simulink model "cubli_XYZ_extensive_simulations"  (R2016a)
settings: Solver=VariableStepAuto  StartTime=0.0  StopTime=10  FixedStep=0.001  RelTol=1e-3
values from neighbouring files (symbols this model uses):
  a = 0.15    [init.m]
  M = 2.5    [init.m]    (also in skew.m = [0 -z y)
  m = 0.204    [init.m]
  s = size(delta_i)    [accessibility_test.m]    (also in observability_test.m = size(delta_i,1))
  state0 = get_equilibrium(0, -pi/4, pi/2, f, state)    [init.m]
undefined symbols (not defined in the file or in its folder): X, Y, Z
libraries: sm_lib x15, nesl_utility x13
(part 7 of 9)

== matlab function cubli_XYZ_extensive_simulations/Cubli/Controller/LQR at equilibrium ==
  data: state input; Q input; R input; u output; theta parameter; state0 parameter
 function u = nic_fnc(state, Q, R, theta, state0)

 %% persistent variables
persistent K_lqr state_eq

 %% lqr cannot be used AS IS in matlab functions
coder.extrinsic('lqr');
coder.extrinsic('ctrbf');

 %% initialize persistent variables
if isempty (K_lqr)
    K_lqr = zeros(3,9);
    state_eq = zeros(9,1);
    K = zeros(3,8);
    Aalt = zeros(9);
    Q_lqr = zeros(9);
    Balt = zeros(9,3);
    
    % equilibrium state
    state_eq = angles(theta, state0);
    
    % linearize around equilibrium
    th1 = state_eq(1);
    th2 = state_eq(2);
    th3 = state_eq(3);
    th1dot = state_eq(4);
    th2dot = state_eq(5);
    th3dot = state_eq(6);
    qxdot = state_eq(7);
    qydot = state_eq(8);
    qzdot = state_eq(9);
    u1 = 0;
    u2 = 0;
    u3 = 0;
    
    % evaluate A and B s.t. dx_dot = A * dx + B * du
    A = [
         0, 0, 0, 1, 0, 0, 0, 0, 0
         0, 0, 0, 0, 1, 0, 0, 0, 0
         0, 0, 0, 0, 0, 1, 0, 0, 0
         (5234057499985498930356104062315637394898944*cos(th1) + 5234057499985498930356104062315637394898944*cos(th2)*sin(th1)*sin(th3) + 5234057499985498930356104062315637394898944*cos(th2)*cos(th3)*sin(th1))/(140800205444266547517405832452217960942325*cos(th2)),                                                                                                                                                                                                                                                                                                                                                                                                                                                                                                                                                                                                                                                                                                                                                                                                                                                                                                                                                                                                                                                                                                                                                                                                                                                                                                                                                                                                                                                                                                                                                                                                                                                                                                                                                                                                                                                                                                                                                                                                                                                                                                                                                                                                                                                                                                                                                                                                                                                                                                                                                                                                                                                                                                                                                                                                                                                                                                                                                                                                                                                                                                                                                                                                                                                                                                                                                                                                                                                                                                                                                                                                                                                                                                                                                                                                                                                                                                                                                                                                                                                                                                                                                                                                                                                                                                                                                                                                                                                                                                                                                                                                                                                                                                                                                                                                                                                                                                                                                                                          (37208574363983751213784670214039629987840*th1dot^2*cos(2*th2) + 5234057499985498930356104062315637394898944*cos(th1)*sin(th2)*sin(th3) + 140800205444266547517405832452217960942325*th1dot*th2dot*cos(th2) - 795598339977096578581794905915392000000*qxdot*th1dot*sin(th2) + 795598339977096578581794905915392000000*qzdot*th1dot*sin(th2) - 37208574363983751213784670214039629987840*th1dot*th3dot*sin(th2) - 74417148727967502427569340428079259975680*th1dot^2*cos(th2)^2*cos(th3)^2 + 74417148727967502427569340428079259975680*th1dot^2*cos(th3)^2*sin(th2)^2 + 5234057499985498930356104062315637394898944*cos(th1)*cos(th3)*sin(th2) + 1419410730694772925795933922925238500000*qxdot*th1dot*cos(th2)*sin(th3) - 795598339977096578581794905915392000000*qydot*th1dot*cos(th2)*sin(th3) - 37208574363983751213784670214039629987840*th1dot*th2dot*cos(th3)*sin(th2) - 74417148727967502427569340428079259975680*th1dot*th3dot*cos(th2)*sin(th3) + 37208574363983751213784670214039629987840*th1dot*th2dot*sin(th2)*sin(th3) + 795598339977096578581794905915392000000*qxdot*th1dot*cos(th3)^2*sin(th2) + 795598339977096578581794905915392000000*qydot*th1dot*cos(th3)^2*sin(th2) - 1591196679954193157163589811830784000000*qzdot*th1dot*cos(th3)^2*sin(th2) + 74417148727967502427569340428079259975680*th1dot*th3dot*cos(th3)^2*sin(th2) - 74417148727967502427569340428079259975680*th1dot^2*cos(th2)*cos(th3)*sin(th2) - 74417148727967502427569340428079259975680*th1dot^2*cos(th2)*sin(th2)*sin(th3) - 795598339977096578581794905915392000000*qxdot*th1dot*cos(th2)*cos(th3) + 1419410730694772925795933922925238500000*qydot*th1dot*cos(th2)*cos(th3) - 74417148727967502427569340428079259975680*th1dot*th3dot*cos(th2)*cos(th3) - 74417148727967502427569340428079259975680*th1dot*th2dot*cos(th2)*cos(th3)*sin(th3) + 795598339977096578581794905915392000000*qxdot*th1dot*cos(th3)*sin(th2)*sin(th3) - 795598339977096578581794905915392000000*qydot*th1dot*cos(th3)*sin(th2)*sin(th3))/(140800205444266547517405832452217960942325*cos(th2)) - (sin(th2)*(37208574363983751213784670214039629987840*th1dot^2*cos(th3) - 5234057499985498930356104062315637394898944*sin(th1) - 37208574363983751213784670214039629987840*th2dot^2*cos(th3) + 37208574363983751213784670214039629987840*th3dot^2*cos(th3) + 37208574363983751213784670214039629987840*th1dot^2*sin(th3) - 37208574363983751213784670214039629987840*th2dot^2*sin(th3) + 37208574363983751213784670214039629987840*th3dot^2*sin(th3) - 795598339977096578581794905915392000000*qydot*th2dot + 1419410730694772925795933922925238500000*qzdot*th2dot + 140800205444266547517405832452217960942325*th2dot*th3dot - 18604287181991875606892335107019814993920*th1dot^2*sin(2*th2) - 795598339977096578581794905915392000000*qxdot*th1dot*cos(th2) + 795598339977096578581794905915392000000*qxdot*th3dot*cos(th3) - 1419410730694772925795933922925238500000*qydot*th3dot*cos(th3) + 795598339977096578581794905915392000000*qzdot*th1dot*cos(th2) - 37208574363983751213784670214039629987840*th1dot*th3dot*cos(th2) - 1419410730694772925795933922925238500000*qxdot*th3dot*sin(th3) + 795598339977096578581794905915392000000*qydot*th3dot*sin(th3) - 140800205444266547517405832452217960942325*th1dot*th2dot*sin(th2) - 37208574363983751213784670214039629987840*th1dot^2*cos(th2)^2*cos(th3) - 37208574363983751213784670214039629987840*th1dot^2*cos(th2)^2*sin(th3) - 795598339977096578581794905915392000000*qxdot*th2dot*cos(th3)^2 + 795598339977096578581794905915392000000*qydot*th2dot*cos(th3)^2 + 397799169988548289290897452957696000000*qxdot*th2dot*sin(2*th3) + 397799169988548289290897452957696000000*qydot*th2dot*sin(2*th3) - 795598339977096578581794905915392000000*qzdot*th2dot*sin(2*th3) + 37208574363983751213784670214039629987840*th2dot*th3dot*sin(2*th3) + 5234057499985498930356104062315637394898944*cos(th1)*cos(th2)*cos(th3) + 5234057499985498930356104062315637394898944*cos(th1)*cos(th2)*sin(th3) + 795598339977096578581794905915392000000*qxdot*th1dot*cos(th3)*sin(th2) - 1419410730694772925795933922925238500000*qydot*th1dot*cos(th3)*sin(th2) + 37208574363983751213784670214039629987840*th1dot*th2dot*cos(th2)*sin(th3) + 74417148727967502427569340428079259975680*th1dot*th3dot*cos(th3)*sin(th2) - 1419410730694772925795933922925238500000*qxdot*th1dot*sin(th2)*sin(th3) + 795598339977096578581794905915392000000*qydot*th1dot*sin(th2)*sin(th3) + 74417148727967502427569340428079259975680*th1dot*th3dot*sin(th2)*sin(th3) + 74417148727967502427569340428079259975680*th1dot^2*cos(th2)*cos(th3)^2*sin(th2) + 795598339977096578581794905915392000000*qxdot*th1dot*cos(th2)*cos(th3)^2 + 795598339977096578581794905915392000000*qydot*th1dot*cos(th2)*cos(th3)^2 - 1591196679954193157163589811830784000000*qzdot*th1dot*cos(th2)*cos(th3)^2 + 74417148727967502427569340428079259975680*th1dot*th3dot*cos(th2)*cos(th3)^2 - 37208574363983751213784670214039629987840*th1dot*th2dot*cos(th2)*cos(th3) + 795598339977096578581794905915392000000*qxdot*th1dot*cos(th2)*cos(th3)*sin(th3) - 795598339977096578581794905915392000000*qydot*th1dot*cos(th2)*cos(th3)*sin(th3) + 74417148727967502427569340428079259975680*th1dot*th2dot*cos(th3)*sin(th2)*sin(th3)))/(140800205444266547517405832452217960942325*cos(th2)^2) - (11529215046068469760000*u1*sin(th2)*(173808361171031714041*cos(th3) - 97421867139278569472*sin(th3)))/(50688073959935957106266099682798465939237*cos(th2)^2) - (11529215046068469760000*u2*sin(th2)*(97421867139278569472*cos(th3) - 173808361171031714041*sin(th3)))/(50688073959935957106266099682798465939237*cos(th2)^2) - (1123197656438253912603716965936891166720000*2^(1/2)*u3*cos(th3 + pi/4)*sin(th2))/(50688073959935957106266099682798465939237*cos(th2)^2),                                                                                                                                                                                                                                                                                                                                                                                                                                                                                                                                                                                                                                                                                                                                                                                                                                                                                                                                                                                                                                                                                                                                                                                                                                                                                                                                                                                                                                                                                                                    (11529215046068469760000*u1*(97421867139278569472*cos(th3) + 173808361171031714041*sin(th3)))/(50688073959935957106266099682798465939237*cos(th2)) - (37208574363983751213784670214039629987840*th1dot^2*cos(th3) - 37208574363983751213784670214039629987840*th2dot^2*cos(th3) + 37208574363983751213784670214039629987840*th3dot^2*cos(th3) - 37208574363983751213784670214039629987840*th1dot^2*sin(th3) + 37208574363983751213784670214039629987840*th2dot^2*sin(th3) - 37208574363983751213784670214039629987840*th3dot^2*sin(th3) - 1419410730694772925795933922925238500000*qxdot*th3dot*cos(th3) + 795598339977096578581794905915392000000*qydot*th3dot*cos(th3) - 795598339977096578581794905915392000000*qxdot*th3dot*sin(th3) + 1419410730694772925795933922925238500000*qydot*th3dot*sin(th3) - 37208574363983751213784670214039629987840*th1dot^2*cos(th2)^2*cos(th3) + 37208574363983751213784670214039629987840*th1dot^2*cos(th2)^2*sin(th3) + 795598339977096578581794905915392000000*qxdot*th2dot*cos(2*th3) + 795598339977096578581794905915392000000*qydot*th2dot*cos(2*th3) - 1591196679954193157163589811830784000000*qzdot*th2dot*cos(2*th3) + 74417148727967502427569340428079259975680*th2dot*th3dot*cos(2*th3) + 5234057499985498930356104062315637394898944*cos(th1)*cos(th2)*cos(th3) - 5234057499985498930356104062315637394898944*cos(th1)*cos(th2)*sin(th3) - 1419410730694772925795933922925238500000*qxdot*th1dot*cos(th3)*sin(th2) + 1591196679954193157163589811830784000000*qxdot*th2dot*cos(th3)*sin(th3) + 795598339977096578581794905915392000000*qydot*th1dot*cos(th3)*sin(th2) - 1591196679954193157163589811830784000000*qydot*th2dot*cos(th3)*sin(th3) + 37208574363983751213784670214039629987840*th1dot*th2dot*cos(th2)*sin(th3) + 74417148727967502427569340428079259975680*th1dot*th3dot*cos(th3)*sin(th2) - 795598339977096578581794905915392000000*qxdot*th1dot*sin(th2)*sin(th3) + 1419410730694772925795933922925238500000*qydot*th1dot*sin(th2)*sin(th3) - 74417148727967502427569340428079259975680*th1dot*th3dot*sin(th2)*sin(th3) + 795598339977096578581794905915392000000*qxdot*th1dot*cos(th2)*cos(th3)^2 - 795598339977096578581794905915392000000*qydot*th1dot*cos(th2)*cos(th3)^2 - 795598339977096578581794905915392000000*qxdot*th1dot*cos(th2)*sin(th3)^2 + 795598339977096578581794905915392000000*qydot*th1dot*cos(th2)*sin(th3)^2 + 74417148727967502427569340428079259975680*th1dot*th2dot*cos(th3)^2*sin(th2) - 74417148727967502427569340428079259975680*th1dot*th2dot*sin(th2)*sin(th3)^2 + 37208574363983751213784670214039629987840*th1dot*th2dot*cos(th2)*cos(th3) - 148834297455935004855138680856158519951360*th1dot^2*cos(th2)*cos(th3)*sin(th2)*sin(th3) - 1591196679954193157163589811830784000000*qxdot*th1dot*cos(th2)*cos(th3)*sin(th3) - 1591196679954193157163589811830784000000*qydot*th1dot*cos(th2)*cos(th3)*sin(th3) + 3182393359908386314327179623661568000000*qzdot*th1dot*cos(th2)*cos(th3)*sin(th3) - 148834297455935004855138680856158519951360*th1dot*th3dot*cos(th2)*cos(th3)*sin(th3))/(140800205444266547517405832452217960942325*cos(th2)) + (11529215046068469760000*u2*(173808361171031714041*cos(th3) + 97421867139278569472*sin(th3)))/(50688073959935957106266099682798465939237*cos(th2)) + (1123197656438253912603716965936891166720000*2^(1/2)*u3*sin(th3 + pi/4))/(50688073959935957106266099682798465939237*cos(th2)),                                                                                                                                                                                                                                                                                                                                                                                                                                 -(795598339977096578581794905915392000000*qzdot*cos(th2) - 795598339977096578581794905915392000000*qxdot*cos(th2) - 37208574363983751213784670214039629987840*th1dot*sin(2*th2) + 74417148727967502427569340428079259975680*th1dot*cos(th3) - 37208574363983751213784670214039629987840*th3dot*cos(th2) + 74417148727967502427569340428079259975680*th1dot*sin(th3) - 140800205444266547517405832452217960942325*th2dot*sin(th2) - 37208574363983751213784670214039629987840*th2dot*cos(th2)*cos(th3) + 795598339977096578581794905915392000000*qxdot*cos(th3)*sin(th2) - 1419410730694772925795933922925238500000*qydot*cos(th3)*sin(th2) + 37208574363983751213784670214039629987840*th2dot*cos(th2)*sin(th3) + 74417148727967502427569340428079259975680*th3dot*cos(th3)*sin(th2) - 1419410730694772925795933922925238500000*qxdot*sin(th2)*sin(th3) + 795598339977096578581794905915392000000*qydot*sin(th2)*sin(th3) + 74417148727967502427569340428079259975680*th3dot*sin(th2)*sin(th3) + 795598339977096578581794905915392000000*qxdot*cos(th2)*cos(th3)^2 + 795598339977096578581794905915392000000*qydot*cos(th2)*cos(th3)^2 - 1591196679954193157163589811830784000000*qzdot*cos(th2)*cos(th3)^2 - 74417148727967502427569340428079259975680*th1dot*cos(th2)^2*cos(th3) + 74417148727967502427569340428079259975680*th3dot*cos(th2)*cos(th3)^2 - 74417148727967502427569340428079259975680*th1dot*cos(th2)^2*sin(th3) + 795598339977096578581794905915392000000*qxdot*cos(th2)*cos(th3)*sin(th3) - 795598339977096578581794905915392000000*qydot*cos(th2)*cos(th3)*sin(th3) + 74417148727967502427569340428079259975680*th2dot*cos(th3)*sin(th2)*sin(th3) + 148834297455935004855138680856158519951360*th1dot*cos(th2)*cos(th3)^2*sin(th2))/(140800205444266547517405832452217960942325*cos(th2)),                                                                                                                                                                                                                                                                                                                                                                                                                                                                                                                                                                                                                                                                                                                                                                 -(1419410730694772925795933922925238500000*qzdot - 795598339977096578581794905915392000000*qydot + 140800205444266547517405832452217960942325*th3dot - 795598339977096578581794905915392000000*qxdot*cos(th3)^2 + 795598339977096578581794905915392000000*qydot*cos(th3)^2 + 397799169988548289290897452957696000000*qxdot*sin(2*th3) + 397799169988548289290897452957696000000*qydot*sin(2*th3) - 795598339977096578581794905915392000000*qzdot*sin(2*th3) + 37208574363983751213784670214039629987840*th3dot*sin(2*th3) - 74417148727967502427569340428079259975680*th2dot*cos(th3) - 140800205444266547517405832452217960942325*th1dot*sin(th2) - 74417148727967502427569340428079259975680*th2dot*sin(th3) - 37208574363983751213784670214039629987840*th1dot*cos(th2)*cos(th3) + 37208574363983751213784670214039629987840*th1dot*cos(th2)*sin(th3) + 74417148727967502427569340428079259975680*th1dot*cos(th3)*sin(th2)*sin(th3))/(140800205444266547517405832452217960942325*cos(th2)),                                                                                                                                                                                                                                                                                                                                                                                                                                                                                  -(140800205444266547517405832452217960942325*th2dot + 37208574363983751213784670214039629987840*th2dot*sin(2*th3) + 795598339977096578581794905915392000000*qxdot*cos(th3) - 1419410730694772925795933922925238500000*qydot*cos(th3) - 37208574363983751213784670214039629987840*th1dot*cos(th2) + 74417148727967502427569340428079259975680*th3dot*cos(th3) - 1419410730694772925795933922925238500000*qxdot*sin(th3) + 795598339977096578581794905915392000000*qydot*sin(th3) + 74417148727967502427569340428079259975680*th3dot*sin(th3) + 74417148727967502427569340428079259975680*th1dot*cos(th3)*sin(th2) + 74417148727967502427569340428079259975680*th1dot*sin(th2)*sin(th3) + 74417148727967502427569340428079259975680*th1dot*cos(th2)*cos(th3)^2)/(140800205444266547517405832452217960942325*cos(th2)),                                                                                                                                                                                                                                                                                                                                -(397799169988548289290897452957696000000*th2dot*sin(2*th3) - 795598339977096578581794905915392000000*th2dot*cos(th3)^2 - 795598339977096578581794905915392000000*th1dot*cos(th2) + 795598339977096578581794905915392000000*th3dot*cos(th3) - 1419410730694772925795933922925238500000*th3dot*sin(th3) + 795598339977096578581794905915392000000*th1dot*cos(th3)*sin(th2) - 1419410730694772925795933922925238500000*th1dot*sin(th2)*sin(th3) + 795598339977096578581794905915392000000*th1dot*cos(th2)*cos(th3)^2 + 795598339977096578581794905915392000000*th1dot*cos(th2)*cos(th3)*sin(th3))/(140800205444266547517405832452217960942325*cos(th2)),                                                                                                                                                                                                                                                                                                                                -(795598339977096578581794905915392000000*th2dot*cos(th3)^2 - 795598339977096578581794905915392000000*th2dot + 397799169988548289290897452957696000000*th2dot*sin(2*th3) - 1419410730694772925795933922925238500000*th3dot*cos(th3) + 795598339977096578581794905915392000000*th3dot*sin(th3) - 1419410730694772925795933922925238500000*th1dot*cos(th3)*sin(th2) + 795598339977096578581794905915392000000*th1dot*sin(th2)*sin(th3) + 795598339977096578581794905915392000000*th1dot*cos(th2)*cos(th3)^2 - 795598339977096578581794905915392000000*th1dot*cos(th2)*cos(th3)*sin(th3))/(140800205444266547517405832452217960942325*cos(th2)),                                                                                                                                                                                                                                                                                                                     -(1419410730694772925795933922925238500000*th2dot - 795598339977096578581794905915392000000*th2dot*sin(2*th3) + 795598339977096578581794905915392000000*th1dot*cos(th2) - 1591196679954193157163589811830784000000*th1dot*cos(th2)*cos(th3)^2)/(140800205444266547517405832452217960942325*cos(th2))
         (68520719092170281189376*cos(th2)*sin(th1)*sin(th3))/1843260477247944264925 - (68520719092170281189376*sin(th1)*sin(th2))/1843260477247944264925 - (68520719092170281189376*cos(th2)*cos(th3)*sin(th1))/1843260477247944264925,                                                                                                                                                                                                                                                                                                                                                                                                                                                                                                                                                                                                                                                                                                                                                                                                                                                                                                                                                                                                                                                                                                                                                                                                                                                                                                                                                                                                                                                                                                                                                                                                                                                                                                                                                                                                                                                                                                                                                                                                                                                                                                                                                                                                                                                                                                                                                                                                                                                                                                                                                                                                                                                                                                                                                                                                                                                                                                                                                                                                                                                                                                                                                                                                                                                                                                                                                                                                                                                                                                                                                                                                                                                                                                                                                                                                                                                                                                                                                                                                                                                                                                                                                                                                                                                                                                                                                                                                                                                                                                                                                                                                                                                                                                                                                                                                                                                                                                                                                                                                                                                                                                                                                                                                                                                                                                                                                                                                                                                                                                                                                                                                                                                                                                                                                                                                                                                                                                                                                                                                                                                                                                                                                                                                                                                                                                                                                                                                                                                                                                                                                                                                                                                                                                                                                                                                                                                                                                                                                                                                                                                                                                                                                                                                                                                                                                                                                                                                                                                                                                                                                                                                                                                                                                                                                                                                                                                                                                                                                                                                                                                                                                                                                                                                                                                                                                                       (68520719092170281189376*cos(th1)*cos(th2))/1843260477247944264925 + (68520719092170281189376*cos(th1)*sin(th2)*sin(th3))/1843260477247944264925 - (97421867139278569472*th1dot*th2dot*cos(th2))/368652095449588852985 + (31823933599083863143271796236615680000*qxdot*th1dot*sin(th2))/5632008217770661900696233298088718437693 - (56776429227790917031837356917009540000*qzdot*th1dot*sin(th2))/5632008217770661900696233298088718437693 - th1dot*th3dot*sin(th2) - (68520719092170281189376*cos(th1)*cos(th3)*sin(th2))/1843260477247944264925 - (31823933599083863143271796236615680000*qxdot*th1dot*cos(th2)*sin(th3))/5632008217770661900696233298088718437693 + (56776429227790917031837356917009540000*qydot*th1dot*cos(th2)*sin(th3))/5632008217770661900696233298088718437693 + (97421867139278569472*th1dot*th2dot*cos(th3)*sin(th2))/368652095449588852985 - (194843734278557138944*th1dot*th3dot*cos(th2)*sin(th3))/368652095449588852985 + (97421867139278569472*th1dot*th2dot*sin(th2)*sin(th3))/368652095449588852985 - (194843734278557138944*th1dot^2*cos(th2)^2*cos(th3)*sin(th3))/368652095449588852985 + (194843734278557138944*th1dot^2*cos(th3)*sin(th2)^2*sin(th3))/368652095449588852985 + (194843734278557138944*th1dot*th2dot*cos(th2)*cos(th3)^2)/368652095449588852985 - (31823933599083863143271796236615680000*qxdot*th1dot*cos(th3)^2*sin(th2))/5632008217770661900696233298088718437693 + (31823933599083863143271796236615680000*qydot*th1dot*cos(th3)^2*sin(th2))/5632008217770661900696233298088718437693 + (389687468557114277888*th1dot^2*cos(th2)*cos(th3)*sin(th2))/368652095449588852985 - (389687468557114277888*th1dot^2*cos(th2)*sin(th2)*sin(th3))/368652095449588852985 - (56776429227790917031837356917009540000*qxdot*th1dot*cos(th2)*cos(th3))/5632008217770661900696233298088718437693 + (31823933599083863143271796236615680000*qydot*th1dot*cos(th2)*cos(th3))/5632008217770661900696233298088718437693 + (194843734278557138944*th1dot*th3dot*cos(th2)*cos(th3))/368652095449588852985 + (31823933599083863143271796236615680000*qxdot*th1dot*cos(th3)*sin(th2)*sin(th3))/5632008217770661900696233298088718437693 + (31823933599083863143271796236615680000*qydot*th1dot*cos(th3)*sin(th2)*sin(th3))/5632008217770661900696233298088718437693 - (63647867198167726286543592473231360000*qzdot*th1dot*cos(th3)*sin(th2)*sin(th3))/5632008217770661900696233298088718437693 + (194843734278557138944*th1dot*th3dot*cos(th3)*sin(th2)*sin(th3))/368652095449588852985,                                                                                                                                                                                                                                                                                                                                                                                                                                                               (56776429227790917031837356917009540000*qydot*th3dot*cos(th3))/5632008217770661900696233298088718437693 - (97421867139278569472*th3dot^2*cos(th3))/368652095449588852985 - u1*((2003873972745561633640040521298775900160000*cos(th3))/50688073959935957106266099682798465939237 - (1123197656438253912603716965936891166720000*sin(th3))/50688073959935957106266099682798465939237) - u2*((1123197656438253912603716965936891166720000*cos(th3))/50688073959935957106266099682798465939237 - (2003873972745561633640040521298775900160000*sin(th3))/50688073959935957106266099682798465939237) - (97421867139278569472*th1dot^2*sin(th3))/368652095449588852985 - (97421867139278569472*th3dot^2*sin(th3))/368652095449588852985 - (1123197656438253912603716965936891166720000*2^(1/2)*u3*cos(th3 + pi/4))/50688073959935957106266099682798465939237 - (31823933599083863143271796236615680000*qxdot*th3dot*cos(th3))/5632008217770661900696233298088718437693 - (97421867139278569472*th1dot^2*cos(th3))/368652095449588852985 + (56776429227790917031837356917009540000*qxdot*th3dot*sin(th3))/5632008217770661900696233298088718437693 - (31823933599083863143271796236615680000*qydot*th3dot*sin(th3))/5632008217770661900696233298088718437693 + (194843734278557138944*th1dot^2*cos(th2)^2*cos(th3))/368652095449588852985 + (194843734278557138944*th1dot^2*cos(th2)^2*sin(th3))/368652095449588852985 + (31823933599083863143271796236615680000*qxdot*th2dot*cos(2*th3))/5632008217770661900696233298088718437693 - (31823933599083863143271796236615680000*qydot*th2dot*cos(2*th3))/5632008217770661900696233298088718437693 - (68520719092170281189376*cos(th1)*cos(th2)*cos(th3))/1843260477247944264925 - (68520719092170281189376*cos(th1)*cos(th2)*sin(th3))/1843260477247944264925 - (31823933599083863143271796236615680000*qxdot*th1dot*cos(th3)*sin(th2))/5632008217770661900696233298088718437693 - (63647867198167726286543592473231360000*qxdot*th2dot*cos(th3)*sin(th3))/5632008217770661900696233298088718437693 + (56776429227790917031837356917009540000*qydot*th1dot*cos(th3)*sin(th2))/5632008217770661900696233298088718437693 - (63647867198167726286543592473231360000*qydot*th2dot*cos(th3)*sin(th3))/5632008217770661900696233298088718437693 + (127295734396335452573087184946462720000*qzdot*th2dot*cos(th3)*sin(th3))/5632008217770661900696233298088718437693 + (97421867139278569472*th1dot*th2dot*cos(th2)*sin(th3))/368652095449588852985 - (194843734278557138944*th1dot*th3dot*cos(th3)*sin(th2))/368652095449588852985 - (389687468557114277888*th2dot*th3dot*cos(th3)*sin(th3))/368652095449588852985 + (56776429227790917031837356917009540000*qxdot*th1dot*sin(th2)*sin(th3))/5632008217770661900696233298088718437693 - (31823933599083863143271796236615680000*qydot*th1dot*sin(th2)*sin(th3))/5632008217770661900696233298088718437693 - (194843734278557138944*th1dot*th3dot*sin(th2)*sin(th3))/368652095449588852985 - (194843734278557138944*th1dot^2*cos(th2)*cos(th3)^2*sin(th2))/368652095449588852985 + (194843734278557138944*th1dot^2*cos(th2)*sin(th2)*sin(th3)^2)/368652095449588852985 - (31823933599083863143271796236615680000*qxdot*th1dot*cos(th2)*cos(th3)^2)/5632008217770661900696233298088718437693 - (31823933599083863143271796236615680000*qydot*th1dot*cos(th2)*cos(th3)^2)/5632008217770661900696233298088718437693 + (63647867198167726286543592473231360000*qzdot*th1dot*cos(th2)*cos(th3)^2)/5632008217770661900696233298088718437693 - (194843734278557138944*th1dot*th3dot*cos(th2)*cos(th3)^2)/368652095449588852985 + (31823933599083863143271796236615680000*qxdot*th1dot*cos(th2)*sin(th3)^2)/5632008217770661900696233298088718437693 + (31823933599083863143271796236615680000*qydot*th1dot*cos(th2)*sin(th3)^2)/5632008217770661900696233298088718437693 - (63647867198167726286543592473231360000*qzdot*th1dot*cos(th2)*sin(th3)^2)/5632008217770661900696233298088718437693 + (194843734278557138944*th1dot*th3dot*cos(th2)*sin(th3)^2)/368652095449588852985 - (97421867139278569472*th1dot*th2dot*cos(th2)*cos(th3))/368652095449588852985 - (63647867198167726286543592473231360000*qxdot*th1dot*cos(th2)*cos(th3)*sin(th3))/5632008217770661900696233298088718437693 + (63647867198167726286543592473231360000*qydot*th1dot*cos(th2)*cos(th3)*sin(th3))/5632008217770661900696233298088718437693 - (389687468557114277888*th1dot*th2dot*cos(th3)*sin(th2)*sin(th3))/368652095449588852985,                                                              (56776429227790917031837356917009540000*qzdot*cos(th2))/5632008217770661900696233298088718437693 - (31823933599083863143271796236615680000*qxdot*cos(th2))/5632008217770661900696233298088718437693 + (194843734278557138944*th1dot*cos(th3))/368652095449588852985 + th3dot*cos(th2) - (194843734278557138944*th1dot*sin(th3))/368652095449588852985 - (97421867139278569472*th2dot*sin(th2))/368652095449588852985 - (97421867139278569472*th2dot*cos(th2)*cos(th3))/368652095449588852985 - (56776429227790917031837356917009540000*qxdot*cos(th3)*sin(th2))/5632008217770661900696233298088718437693 + (31823933599083863143271796236615680000*qydot*cos(th3)*sin(th2))/5632008217770661900696233298088718437693 - (97421867139278569472*th2dot*cos(th2)*sin(th3))/368652095449588852985 + (194843734278557138944*th3dot*cos(th3)*sin(th2))/368652095449588852985 - (31823933599083863143271796236615680000*qxdot*sin(th2)*sin(th3))/5632008217770661900696233298088718437693 + (56776429227790917031837356917009540000*qydot*sin(th2)*sin(th3))/5632008217770661900696233298088718437693 - (194843734278557138944*th3dot*sin(th2)*sin(th3))/368652095449588852985 + (31823933599083863143271796236615680000*qxdot*cos(th2)*cos(th3)^2)/5632008217770661900696233298088718437693 - (31823933599083863143271796236615680000*qydot*cos(th2)*cos(th3)^2)/5632008217770661900696233298088718437693 - (389687468557114277888*th1dot*cos(th2)^2*cos(th3))/368652095449588852985 + (389687468557114277888*th1dot*cos(th2)^2*sin(th3))/368652095449588852985 + (194843734278557138944*th2dot*cos(th3)^2*sin(th2))/368652095449588852985 - (31823933599083863143271796236615680000*qxdot*cos(th2)*cos(th3)*sin(th3))/5632008217770661900696233298088718437693 - (31823933599083863143271796236615680000*qydot*cos(th2)*cos(th3)*sin(th3))/5632008217770661900696233298088718437693 + (63647867198167726286543592473231360000*qzdot*cos(th2)*cos(th3)*sin(th3))/5632008217770661900696233298088718437693 - (194843734278557138944*th3dot*cos(th2)*cos(th3)*sin(th3))/368652095449588852985 - (389687468557114277888*th1dot*cos(th2)*cos(th3)*sin(th2)*sin(th3))/368652095449588852985,                                                                                                                                                                                                                                                                                                                                                                                                                                                                                                                                                                                                                                  (31823933599083863143271796236615680000*qzdot)/5632008217770661900696233298088718437693 - (31823933599083863143271796236615680000*qydot)/5632008217770661900696233298088718437693 - (97421867139278569472*th3dot)/368652095449588852985 + (31823933599083863143271796236615680000*qxdot*cos(th3)^2)/5632008217770661900696233298088718437693 + (31823933599083863143271796236615680000*qydot*cos(th3)^2)/5632008217770661900696233298088718437693 - (63647867198167726286543592473231360000*qzdot*cos(th3)^2)/5632008217770661900696233298088718437693 + (194843734278557138944*th3dot*cos(th3)^2)/368652095449588852985 + (15911966799541931571635898118307840000*qxdot*sin(2*th3))/5632008217770661900696233298088718437693 - (15911966799541931571635898118307840000*qydot*sin(2*th3))/5632008217770661900696233298088718437693 - (97421867139278569472*th1dot*sin(th2))/368652095449588852985 - (97421867139278569472*th1dot*cos(th2)*cos(th3))/368652095449588852985 - (97421867139278569472*th1dot*cos(th2)*sin(th3))/368652095449588852985 + (194843734278557138944*th1dot*cos(th3)^2*sin(th2))/368652095449588852985,                                                                                                                                                                                                                                                                                                                                                                              (194843734278557138944*th2dot*cos(th3)^2)/368652095449588852985 - (97421867139278569472*th2dot)/368652095449588852985 - (56776429227790917031837356917009540000*qxdot*cos(th3))/5632008217770661900696233298088718437693 + (31823933599083863143271796236615680000*qydot*cos(th3))/5632008217770661900696233298088718437693 + th1dot*cos(th2) + (194843734278557138944*th3dot*cos(th3))/368652095449588852985 - (31823933599083863143271796236615680000*qxdot*sin(th3))/5632008217770661900696233298088718437693 + (56776429227790917031837356917009540000*qydot*sin(th3))/5632008217770661900696233298088718437693 - (194843734278557138944*th3dot*sin(th3))/368652095449588852985 + (194843734278557138944*th1dot*cos(th3)*sin(th2))/368652095449588852985 - (194843734278557138944*th1dot*sin(th2)*sin(th3))/368652095449588852985 - (194843734278557138944*th1dot*cos(th2)*cos(th3)*sin(th3))/368652095449588852985, (31823933599083863143271796236615680000*th2dot*cos(th3)^2)/5632008217770661900696233298088718437693 + (15911966799541931571635898118307840000*th2dot*sin(2*th3))/5632008217770661900696233298088718437693 - (31823933599083863143271796236615680000*th1dot*cos(th2))/5632008217770661900696233298088718437693 - (56776429227790917031837356917009540000*th3dot*cos(th3))/5632008217770661900696233298088718437693 - (31823933599083863143271796236615680000*th3dot*sin(th3))/5632008217770661900696233298088718437693 - (56776429227790917031837356917009540000*th1dot*cos(th3)*sin(th2))/5632008217770661900696233298088718437693 - (31823933599083863143271796236615680000*th1dot*sin(th2)*sin(th3))/5632008217770661900696233298088718437693 + (31823933599083863143271796236615680000*th1dot*cos(th2)*cos(th3)^2)/5632008217770661900696233298088718437693 - (31823933599083863143271796236615680000*th1dot*cos(th2)*cos(th3)*sin(th3))/5632008217770661900696233298088718437693, (31823933599083863143271796236615680000*th2dot*cos(th3)^2)/5632008217770661900696233298088718437693 - (31823933599083863143271796236615680000*th2dot)/5632008217770661900696233298088718437693 - (15911966799541931571635898118307840000*th2dot*sin(2*th3))/5632008217770661900696233298088718437693 + (31823933599083863143271796236615680000*th3dot*cos(th3))/5632008217770661900696233298088718437693 + (56776429227790917031837356917009540000*th3dot*sin(th3))/5632008217770661900696233298088718437693 + (31823933599083863143271796236615680000*th1dot*cos(th3)*sin(th2))/5632008217770661900696233298088718437693 + (56776429227790917031837356917009540000*th1dot*sin(th2)*sin(th3))/5632008217770661900696233298088718437693 - (31823933599083863143271796236615680000*th1dot*cos(th2)*cos(th3)^2)/5632008217770661900696233298088718437693 - (31823933599083863143271796236615680000*th1dot*cos(th2)*cos(th3)*sin(th3))/5632008217770661900696233298088718437693,                                                                                                                                                                                                 (31823933599083863143271796236615680000*th2dot)/5632008217770661900696233298088718437693 - (63647867198167726286543592473231360000*th2dot*cos(th3)^2)/5632008217770661900696233298088718437693 + (56776429227790917031837356917009540000*th1dot*cos(th2))/5632008217770661900696233298088718437693 + (63647867198167726286543592473231360000*th1dot*cos(th2)*cos(th3)*sin(th3))/5632008217770661900696233298088718437693
         -(5234057499985498930356104062315637394898944*cos(th1)*sin(th2) + 5234057499985498930356104062315637394898944*cos(th1)*cos(th2)*cos(th3) - 5234057499985498930356104062315637394898944*cos(th1)*cos(th2)*sin(th3))/(140800205444266547517405832452217960942325*cos(th2)), (37208574363983751213784670214039629987840*th1dot^2*sin(th2) - 37208574363983751213784670214039629987840*th2dot^2*sin(th2) - 5234057499985498930356104062315637394898944*cos(th2)*sin(th1) + 5234057499985498930356104062315637394898944*cos(th3)*sin(th1)*sin(th2) - 5234057499985498930356104062315637394898944*sin(th1)*sin(th2)*sin(th3) - 795598339977096578581794905915392000000*qydot*th2dot*cos(th2) + 1419410730694772925795933922925238500000*qzdot*th2dot*cos(th2) + 140800205444266547517405832452217960942325*th2dot*th3dot*cos(th2) + 795598339977096578581794905915392000000*qxdot*th3dot*sin(th2) - 795598339977096578581794905915392000000*qydot*th3dot*sin(th2) - 74417148727967502427569340428079259975680*th1dot^2*cos(th3)^2*sin(th2) + 74417148727967502427569340428079259975680*th2dot^2*cos(th3)^2*sin(th2) - 1591196679954193157163589811830784000000*qxdot*th1dot*cos(2*th2) + 795598339977096578581794905915392000000*qydot*th1dot*cos(2*th2) + 795598339977096578581794905915392000000*qzdot*th1dot*cos(2*th2) - 37208574363983751213784670214039629987840*th1dot*th3dot*cos(2*th2) + 37208574363983751213784670214039629987840*th1dot^2*cos(th2)*cos(th3) - 37208574363983751213784670214039629987840*th2dot^2*cos(th2)*cos(th3) + 37208574363983751213784670214039629987840*th3dot^2*cos(th2)*cos(th3) + 37208574363983751213784670214039629987840*th1dot^2*cos(th2)*sin(th3) - 37208574363983751213784670214039629987840*th2dot^2*cos(th2)*sin(th3) + 37208574363983751213784670214039629987840*th3dot^2*cos(th2)*sin(th3) - 1419410730694772925795933922925238500000*qxdot*th2dot*cos(th3)*sin(th2) - 1419410730694772925795933922925238500000*qxdot*th3dot*cos(th2)*sin(th3) + 795598339977096578581794905915392000000*qydot*th3dot*cos(th2)*sin(th3) + 795598339977096578581794905915392000000*qzdot*th2dot*cos(th3)*sin(th2) + 37208574363983751213784670214039629987840*th2dot*th3dot*cos(th3)*sin(th2) + 1419410730694772925795933922925238500000*qydot*th2dot*sin(th2)*sin(th3) - 795598339977096578581794905915392000000*qzdot*th2dot*sin(th2)*sin(th3) - 37208574363983751213784670214039629987840*th2dot*th3dot*sin(th2)*sin(th3) - 795598339977096578581794905915392000000*qxdot*th2dot*cos(th2)*cos(th3)^2 + 795598339977096578581794905915392000000*qydot*th2dot*cos(th2)*cos(th3)^2 - 74417148727967502427569340428079259975680*th1dot*th2dot*cos(th2)^2*cos(th3) + 74417148727967502427569340428079259975680*th1dot*th2dot*cos(th3)*sin(th2)^2 + 74417148727967502427569340428079259975680*th1dot*th2dot*cos(th2)^2*sin(th3) - 74417148727967502427569340428079259975680*th1dot*th2dot*sin(th2)^2*sin(th3) + 795598339977096578581794905915392000000*qxdot*th1dot*cos(th2)^2*cos(th3)^2 + 795598339977096578581794905915392000000*qydot*th1dot*cos(th2)^2*cos(th3)^2 - 1591196679954193157163589811830784000000*qzdot*th1dot*cos(th2)^2*cos(th3)^2 + 74417148727967502427569340428079259975680*th1dot*th3dot*cos(th2)^2*cos(th3)^2 - 795598339977096578581794905915392000000*qxdot*th1dot*cos(th3)^2*sin(th2)^2 - 795598339977096578581794905915392000000*qydot*th1dot*cos(th3)^2*sin(th2)^2 + 1591196679954193157163589811830784000000*qzdot*th1dot*cos(th3)^2*sin(th2)^2 - 74417148727967502427569340428079259975680*th1dot*th3dot*cos(th3)^2*sin(th2)^2 + 795598339977096578581794905915392000000*qxdot*th3dot*cos(th2)*cos(th3) - 1419410730694772925795933922925238500000*qydot*th3dot*cos(th2)*cos(th3) + 795598339977096578581794905915392000000*qxdot*th1dot*cos(th2)^2*cos(th3)*sin(th3) - 795598339977096578581794905915392000000*qydot*th1dot*cos(th2)^2*cos(th3)*sin(th3) - 795598339977096578581794905915392000000*qxdot*th1dot*cos(th3)*sin(th2)^2*sin(th3) + 795598339977096578581794905915392000000*qydot*th1dot*cos(th3)*sin(th2)^2*sin(th3) + 1591196679954193157163589811830784000000*qxdot*th1dot*cos(th2)*cos(th3)*sin(th2) + 795598339977096578581794905915392000000*qxdot*th2dot*cos(th2)*cos(th3)*sin(th3) + 795598339977096578581794905915392000000*qydot*th2dot*cos(th2)*cos(th3)*sin(th3) - 1591196679954193157163589811830784000000*qzdot*th1dot*cos(th2)*cos(th3)*sin(th2) - 1591196679954193157163589811830784000000*qzdot*th2dot*cos(th2)*cos(th3)*sin(th3) + 74417148727967502427569340428079259975680*th1dot*th3dot*cos(th2)*cos(th3)*sin(th2) + 74417148727967502427569340428079259975680*th2dot*th3dot*cos(th2)*cos(th3)*sin(th3) + 1591196679954193157163589811830784000000*qydot*th1dot*cos(th2)*sin(th2)*sin(th3) - 1591196679954193157163589811830784000000*qzdot*th1dot*cos(th2)*sin(th2)*sin(th3) + 74417148727967502427569340428079259975680*th1dot*th3dot*cos(th2)*sin(th2)*sin(th3) - 148834297455935004855138680856158519951360*th1dot*th2dot*cos(th2)*cos(th3)*sin(th2)*sin(th3))/(140800205444266547517405832452217960942325*cos(th2)) + (11529215046068469760000*u1*(97421867139278569472*sin(th2) + 173808361171031714041*cos(th2)*cos(th3) - 97421867139278569472*cos(th2)*sin(th3)))/(50688073959935957106266099682798465939237*cos(th2)) + (11529215046068469760000*u2*(97421867139278569472*sin(th2) + 97421867139278569472*cos(th2)*cos(th3) - 173808361171031714041*cos(th2)*sin(th3)))/(50688073959935957106266099682798465939237*cos(th2)) + (11529215046068469760000*u3*(173808361171031714041*sin(th2) + 97421867139278569472*cos(th2)*cos(th3) - 97421867139278569472*cos(th2)*sin(th3)))/(50688073959935957106266099682798465939237*cos(th2)) + (sin(th2)*(37208574363983751213784670214039629987840*th2dot^2*cos(th2) - 37208574363983751213784670214039629987840*th1dot^2*cos(th2) - 5234057499985498930356104062315637394898944*sin(th1)*sin(th2) - 140800205444266547517405832452217960942325*th1dot*th2dot + 37208574363983751213784670214039629987840*th1dot^2*sin(th2)*sin(th3) - 37208574363983751213784670214039629987840*th2dot^2*sin(th2)*sin(th3) + 37208574363983751213784670214039629987840*th3dot^2*sin(th2)*sin(th3) + 5234057499985498930356104062315637394898944*cos(th2)*sin(th1)*sin(th3) + 795598339977096578581794905915392000000*qxdot*th1dot*cos(th3) - 795598339977096578581794905915392000000*qxdot*th3dot*cos(th2) - 1419410730694772925795933922925238500000*qydot*th1dot*cos(th3) + 795598339977096578581794905915392000000*qydot*th3dot*cos(th2) + 74417148727967502427569340428079259975680*th1dot*th3dot*cos(th3) - 1419410730694772925795933922925238500000*qxdot*th1dot*sin(th3) + 795598339977096578581794905915392000000*qydot*th1dot*sin(th3) - 795598339977096578581794905915392000000*qydot*th2dot*sin(th2) + 1419410730694772925795933922925238500000*qzdot*th2dot*sin(th2) + 74417148727967502427569340428079259975680*th1dot*th3dot*sin(th3) + 140800205444266547517405832452217960942325*th2dot*th3dot*sin(th2) + 74417148727967502427569340428079259975680*th1dot^2*cos(th2)*cos(th3)^2 - 74417148727967502427569340428079259975680*th2dot^2*cos(th2)*cos(th3)^2 - 795598339977096578581794905915392000000*qxdot*th1dot*sin(2*th2) + 397799169988548289290897452957696000000*qydot*th1dot*sin(2*th2) + 397799169988548289290897452957696000000*qzdot*th1dot*sin(2*th2) + 37208574363983751213784670214039629987840*th1dot*th2dot*sin(2*th3) - 18604287181991875606892335107019814993920*th1dot*th3dot*sin(2*th2) + 37208574363983751213784670214039629987840*th1dot^2*cos(th3)*sin(th2) - 37208574363983751213784670214039629987840*th2dot^2*cos(th3)*sin(th2) + 37208574363983751213784670214039629987840*th3dot^2*cos(th3)*sin(th2) - 5234057499985498930356104062315637394898944*cos(th2)*cos(th3)*sin(th1) + 795598339977096578581794905915392000000*qxdot*th3dot*cos(th3)*sin(th2) - 1419410730694772925795933922925238500000*qydot*th2dot*cos(th2)*sin(th3) - 1419410730694772925795933922925238500000*qydot*th3dot*cos(th3)*sin(th2) + 795598339977096578581794905915392000000*qzdot*th2dot*cos(th2)*sin(th3) + 37208574363983751213784670214039629987840*th2dot*th3dot*cos(th2)*sin(th3) - 1419410730694772925795933922925238500000*qxdot*th3dot*sin(th2)*sin(th3) + 795598339977096578581794905915392000000*qydot*th3dot*sin(th2)*sin(th3) - 795598339977096578581794905915392000000*qxdot*th1dot*cos(th2)^2*cos(th3) + 795598339977096578581794905915392000000*qzdot*th1dot*cos(th2)^2*cos(th3) - 37208574363983751213784670214039629987840*th1dot*th3dot*cos(th2)^2*cos(th3) - 795598339977096578581794905915392000000*qxdot*th2dot*cos(th3)^2*sin(th2) - 795598339977096578581794905915392000000*qydot*th1dot*cos(th2)^2*sin(th3) + 795598339977096578581794905915392000000*qydot*th2dot*cos(th3)^2*sin(th2) + 795598339977096578581794905915392000000*qzdot*th1dot*cos(th2)^2*sin(th3) - 37208574363983751213784670214039629987840*th1dot*th3dot*cos(th2)^2*sin(th3) + 1419410730694772925795933922925238500000*qxdot*th2dot*cos(th2)*cos(th3) - 795598339977096578581794905915392000000*qzdot*th2dot*cos(th2)*cos(th3) - 37208574363983751213784670214039629987840*th2dot*th3dot*cos(th2)*cos(th3) + 795598339977096578581794905915392000000*qxdot*th1dot*cos(th2)*cos(th3)^2*sin(th2) + 795598339977096578581794905915392000000*qydot*th1dot*cos(th2)*cos(th3)^2*sin(th2) - 1591196679954193157163589811830784000000*qzdot*th1dot*cos(th2)*cos(th3)^2*sin(th2) + 74417148727967502427569340428079259975680*th1dot*th2dot*cos(th2)^2*cos(th3)*sin(th3) + 74417148727967502427569340428079259975680*th1dot*th3dot*cos(th2)*cos(th3)^2*sin(th2) - 74417148727967502427569340428079259975680*th1dot*th2dot*cos(th2)*cos(th3)*sin(th2) + 795598339977096578581794905915392000000*qxdot*th2dot*cos(th3)*sin(th2)*sin(th3) + 795598339977096578581794905915392000000*qydot*th2dot*cos(th3)*sin(th2)*sin(th3) - 1591196679954193157163589811830784000000*qzdot*th2dot*cos(th3)*sin(th2)*sin(th3) + 74417148727967502427569340428079259975680*th1dot*th2dot*cos(th2)*sin(th2)*sin(th3) + 74417148727967502427569340428079259975680*th2dot*th3dot*cos(th3)*sin(th2)*sin(th3) + 795598339977096578581794905915392000000*qxdot*th1dot*cos(th2)*cos(th3)*sin(th2)*sin(th3) - 795598339977096578581794905915392000000*qydot*th1dot*cos(th2)*cos(th3)*sin(th2)*sin(th3)))/(140800205444266547517405832452217960942325*cos(th2)^2) - (11529215046068469760000*u1*sin(th2)*(97421867139278569472*cos(th2) - 173808361171031714041*cos(th3)*sin(th2) + 97421867139278569472*sin(th2)*sin(th3)))/(50688073959935957106266099682798465939237*cos(th2)^2) - (11529215046068469760000*u2*sin(th2)*(97421867139278569472*cos(th2) - 97421867139278569472*cos(th3)*sin(th2) + 173808361171031714041*sin(th2)*sin(th3)))/(50688073959935957106266099682798465939237*cos(th2)^2) - (11529215046068469760000*u3*sin(th2)*(173808361171031714041*cos(th2) - 97421867139278569472*cos(th3)*sin(th2) + 97421867139278569472*sin(th2)*sin(th3)))/(50688073959935957106266099682798465939237*cos(th2)^2), (37208574363983751213784670214039629987840*th2dot^2*sin(th2)*sin(th3) - 37208574363983751213784670214039629987840*th1dot^2*sin(th2)*sin(th3) - 37208574363983751213784670214039629987840*th3dot^2*sin(th2)*sin(th3) + 5234057499985498930356104062315637394898944*cos(th2)*sin(th1)*sin(th3) - 1419410730694772925795933922925238500000*qxdot*th1dot*cos(th3) + 795598339977096578581794905915392000000*qydot*th1dot*cos(th3) + 74417148727967502427569340428079259975680*th1dot*th3dot*cos(th3) - 795598339977096578581794905915392000000*qxdot*th1dot*sin(th3) + 1419410730694772925795933922925238500000*qydot*th1dot*sin(th3) - 74417148727967502427569340428079259975680*th1dot*th3dot*sin(th3) + 74417148727967502427569340428079259975680*th1dot*th2dot*cos(2*th3) + 37208574363983751213784670214039629987840*th1dot^2*cos(th3)*sin(th2) - 37208574363983751213784670214039629987840*th2dot^2*cos(th3)*sin(th2) + 37208574363983751213784670214039629987840*th3dot^2*cos(th3)*sin(th2) + 5234057499985498930356104062315637394898944*cos(th2)*cos(th3)*sin(th1) - 1419410730694772925795933922925238500000*qxdot*th2dot*cos(th2)*sin(th3) - 1419410730694772925795933922925238500000*qxdot*th3dot*cos(th3)*sin(th2) + 795598339977096578581794905915392000000*qydot*th3dot*cos(th3)*sin(th2) + 795598339977096578581794905915392000000*qzdot*th2dot*cos(th2)*sin(th3) + 37208574363983751213784670214039629987840*th2dot*th3dot*cos(th2)*sin(th3) - 795598339977096578581794905915392000000*qxdot*th3dot*sin(th2)*sin(th3) + 1419410730694772925795933922925238500000*qydot*th3dot*sin(th2)*sin(th3) - 795598339977096578581794905915392000000*qydot*th1dot*cos(th2)^2*cos(th3) + 795598339977096578581794905915392000000*qzdot*th1dot*cos(th2)^2*cos(th3) - 37208574363983751213784670214039629987840*th1dot*th3dot*cos(th2)^2*cos(th3) + 795598339977096578581794905915392000000*qxdot*th1dot*cos(th2)^2*sin(th3) + 795598339977096578581794905915392000000*qxdot*th2dot*cos(th3)^2*sin(th2) + 795598339977096578581794905915392000000*qydot*th2dot*cos(th3)^2*sin(th2) - 795598339977096578581794905915392000000*qzdot*th1dot*cos(th2)^2*sin(th3) - 1591196679954193157163589811830784000000*qzdot*th2dot*cos(th3)^2*sin(th2) + 37208574363983751213784670214039629987840*th1dot*th3dot*cos(th2)^2*sin(th3) + 74417148727967502427569340428079259975680*th2dot*th3dot*cos(th3)^2*sin(th2) - 795598339977096578581794905915392000000*qxdot*th2dot*sin(th2)*sin(th3)^2 - 795598339977096578581794905915392000000*qydot*th2dot*sin(th2)*sin(th3)^2 + 1591196679954193157163589811830784000000*qzdot*th2dot*sin(th2)*sin(th3)^2 - 74417148727967502427569340428079259975680*th2dot*th3dot*sin(th2)*sin(th3)^2 + 74417148727967502427569340428079259975680*th1dot*th2dot*cos(th2)^2*cos(th3)^2 - 74417148727967502427569340428079259975680*th1dot*th2dot*cos(th2)^2*sin(th3)^2 - 148834297455935004855138680856158519951360*th1dot^2*cos(th2)*cos(th3)*sin(th3) + 148834297455935004855138680856158519951360*th2dot^2*cos(th2)*cos(th3)*sin(th3) - 1419410730694772925795933922925238500000*qydot*th2dot*cos(th2)*cos(th3) + 795598339977096578581794905915392000000*qzdot*th2dot*cos(th2)*cos(th3) + 37208574363983751213784670214039629987840*th2dot*th3dot*cos(th2)*cos(th3) + 795598339977096578581794905915392000000*qxdot*th1dot*cos(th2)*cos(th3)^2*sin(th2) - 795598339977096578581794905915392000000*qydot*th1dot*cos(th2)*cos(th3)^2*sin(th2) - 795598339977096578581794905915392000000*qxdot*th1dot*cos(th2)*sin(th2)*sin(th3)^2 + 795598339977096578581794905915392000000*qydot*th1dot*cos(th2)*sin(th2)*sin(th3)^2 + 74417148727967502427569340428079259975680*th1dot*th2dot*cos(th2)*cos(th3)*sin(th2) + 1591196679954193157163589811830784000000*qxdot*th2dot*cos(th3)*sin(th2)*sin(th3) - 1591196679954193157163589811830784000000*qydot*th2dot*cos(th3)*sin(th2)*sin(th3) + 74417148727967502427569340428079259975680*th1dot*th2dot*cos(th2)*sin(th2)*sin(th3) - 1591196679954193157163589811830784000000*qxdot*th1dot*cos(th2)*cos(th3)*sin(th2)*sin(th3) - 1591196679954193157163589811830784000000*qydot*th1dot*cos(th2)*cos(th3)*sin(th2)*sin(th3) + 3182393359908386314327179623661568000000*qzdot*th1dot*cos(th2)*cos(th3)*sin(th2)*sin(th3) - 148834297455935004855138680856158519951360*th1dot*th3dot*cos(th2)*cos(th3)*sin(th2)*sin(th3))/(140800205444266547517405832452217960942325*cos(th2)) - (11529215046068469760000*u1*(97421867139278569472*cos(th3)*sin(th2) + 173808361171031714041*sin(th2)*sin(th3)))/(50688073959935957106266099682798465939237*cos(th2)) - (11529215046068469760000*u2*(173808361171031714041*cos(th3)*sin(th2) + 97421867139278569472*sin(th2)*sin(th3)))/(50688073959935957106266099682798465939237*cos(th2)) - (11529215046068469760000*u3*(97421867139278569472*cos(th3)*sin(th2) + 97421867139278569472*sin(th2)*sin(th3)))/(50688073959935957106266099682798465939237*cos(th2)), (397799169988548289290897452957696000000*qydot*sin(2*th2) - 795598339977096578581794905915392000000*qxdot*sin(2*th2) - 140800205444266547517405832452217960942325*th2dot + 397799169988548289290897452957696000000*qzdot*sin(2*th2) + 37208574363983751213784670214039629987840*th2dot*sin(2*th3) - 18604287181991875606892335107019814993920*th3dot*sin(2*th2) + 795598339977096578581794905915392000000*qxdot*cos(th3) - 1419410730694772925795933922925238500000*qydot*cos(th3) - 74417148727967502427569340428079259975680*th1dot*cos(th2) + 74417148727967502427569340428079259975680*th3dot*cos(th3) - 1419410730694772925795933922925238500000*qxdot*sin(th3) + 795598339977096578581794905915392000000*qydot*sin(th3) + 74417148727967502427569340428079259975680*th3dot*sin(th3) + 74417148727967502427569340428079259975680*th1dot*cos(th3)*sin(th2) + 74417148727967502427569340428079259975680*th1dot*sin(th2)*sin(th3) - 795598339977096578581794905915392000000*qxdot*cos(th2)^2*cos(th3) + 795598339977096578581794905915392000000*qzdot*cos(th2)^2*cos(th3) + 148834297455935004855138680856158519951360*th1dot*cos(th2)*cos(th3)^2 - 37208574363983751213784670214039629987840*th3dot*cos(th2)^2*cos(th3) - 795598339977096578581794905915392000000*qydot*cos(th2)^2*sin(th3) + 795598339977096578581794905915392000000*qzdot*cos(th2)^2*sin(th3) - 37208574363983751213784670214039629987840*th3dot*cos(th2)^2*sin(th3) - 74417148727967502427569340428079259975680*th2dot*cos(th2)*cos(th3)*sin(th2) + 74417148727967502427569340428079259975680*th2dot*cos(th2)*sin(th2)*sin(th3) + 795598339977096578581794905915392000000*qxdot*cos(th2)*cos(th3)^2*sin(th2) + 795598339977096578581794905915392000000*qydot*cos(th2)*cos(th3)^2*sin(th2) - 1591196679954193157163589811830784000000*qzdot*cos(th2)*cos(th3)^2*sin(th2) + 74417148727967502427569340428079259975680*th2dot*cos(th2)^2*cos(th3)*sin(th3) + 74417148727967502427569340428079259975680*th3dot*cos(th2)*cos(th3)^2*sin(th2) + 795598339977096578581794905915392000000*qxdot*cos(th2)*cos(th3)*sin(th2)*sin(th3) - 795598339977096578581794905915392000000*qydot*cos(th2)*cos(th3)*sin(th2)*sin(th3))/(140800205444266547517405832452217960942325*cos(th2)), (37208574363983751213784670214039629987840*th1dot*sin(2*th3) - 140800205444266547517405832452217960942325*th1dot + 74417148727967502427569340428079259975680*th2dot*cos(th2) - 795598339977096578581794905915392000000*qydot*sin(th2) + 1419410730694772925795933922925238500000*qzdot*sin(th2) + 140800205444266547517405832452217960942325*th3dot*sin(th2) + 1419410730694772925795933922925238500000*qxdot*cos(th2)*cos(th3) - 795598339977096578581794905915392000000*qzdot*cos(th2)*cos(th3) - 37208574363983751213784670214039629987840*th3dot*cos(th2)*cos(th3) - 1419410730694772925795933922925238500000*qydot*cos(th2)*sin(th3) + 795598339977096578581794905915392000000*qzdot*cos(th2)*sin(th3) - 74417148727967502427569340428079259975680*th2dot*cos(th3)*sin(th2) + 37208574363983751213784670214039629987840*th3dot*cos(th2)*sin(th3) - 74417148727967502427569340428079259975680*th2dot*sin(th2)*sin(th3) - 148834297455935004855138680856158519951360*th2dot*cos(th2)*cos(th3)^2 - 795598339977096578581794905915392000000*qxdot*cos(th3)^2*sin(th2) + 795598339977096578581794905915392000000*qydot*cos(th3)^2*sin(th2) - 74417148727967502427569340428079259975680*th1dot*cos(th2)*cos(th3)*sin(th2) + 795598339977096578581794905915392000000*qxdot*cos(th3)*sin(th2)*sin(th3) + 795598339977096578581794905915392000000*qydot*cos(th3)*sin(th2)*sin(th3) - 1591196679954193157163589811830784000000*qzdot*cos(th3)*sin(th2)*sin(th3) + 74417148727967502427569340428079259975680*th1dot*cos(th2)*sin(th2)*sin(th3) + 74417148727967502427569340428079259975680*th3dot*cos(th3)*sin(th2)*sin(th3) + 74417148727967502427569340428079259975680*th1dot*cos(th2)^2*cos(th3)*sin(th3))/(140800205444266547517405832452217960942325*cos(th2)), (795598339977096578581794905915392000000*qydot*cos(th2) - 795598339977096578581794905915392000000*qxdot*cos(th2) - 18604287181991875606892335107019814993920*th1dot*sin(2*th2) + 74417148727967502427569340428079259975680*th1dot*cos(th3) + 74417148727967502427569340428079259975680*th1dot*sin(th3) + 140800205444266547517405832452217960942325*th2dot*sin(th2) - 37208574363983751213784670214039629987840*th2dot*cos(th2)*cos(th3) + 795598339977096578581794905915392000000*qxdot*cos(th3)*sin(th2) - 1419410730694772925795933922925238500000*qydot*cos(th3)*sin(th2) + 37208574363983751213784670214039629987840*th2dot*cos(th2)*sin(th3) + 74417148727967502427569340428079259975680*th3dot*cos(th3)*sin(th2) - 1419410730694772925795933922925238500000*qxdot*sin(th2)*sin(th3) + 795598339977096578581794905915392000000*qydot*sin(th2)*sin(th3) + 74417148727967502427569340428079259975680*th3dot*sin(th2)*sin(th3) - 37208574363983751213784670214039629987840*th1dot*cos(th2)^2*cos(th3) - 37208574363983751213784670214039629987840*th1dot*cos(th2)^2*sin(th3) + 74417148727967502427569340428079259975680*th2dot*cos(th3)*sin(th2)*sin(th3) + 74417148727967502427569340428079259975680*th1dot*cos(th2)*cos(th3)^2*sin(th2))/(140800205444266547517405832452217960942325*cos(th2)),                                                                                -(795598339977096578581794905915392000000*th1dot*sin(2*th2) - 795598339977096578581794905915392000000*th1dot*cos(th3) + 795598339977096578581794905915392000000*th3dot*cos(th2) + 1419410730694772925795933922925238500000*th1dot*sin(th3) - 1419410730694772925795933922925238500000*th2dot*cos(th2)*cos(th3) - 795598339977096578581794905915392000000*th3dot*cos(th3)*sin(th2) + 1419410730694772925795933922925238500000*th3dot*sin(th2)*sin(th3) + 795598339977096578581794905915392000000*th1dot*cos(th2)^2*cos(th3) + 795598339977096578581794905915392000000*th2dot*cos(th3)^2*sin(th2) - 795598339977096578581794905915392000000*th2dot*cos(th3)*sin(th2)*sin(th3) - 795598339977096578581794905915392000000*th1dot*cos(th2)*cos(th3)^2*sin(th2) - 795598339977096578581794905915392000000*th1dot*cos(th2)*cos(th3)*sin(th2)*sin(th3))/(140800205444266547517405832452217960942325*cos(th2)),              (397799169988548289290897452957696000000*th1dot*sin(2*th2) - 1419410730694772925795933922925238500000*th1dot*cos(th3) + 795598339977096578581794905915392000000*th3dot*cos(th2) + 795598339977096578581794905915392000000*th1dot*sin(th3) - 795598339977096578581794905915392000000*th2dot*sin(th2) - 1419410730694772925795933922925238500000*th2dot*cos(th2)*sin(th3) - 1419410730694772925795933922925238500000*th3dot*cos(th3)*sin(th2) + 795598339977096578581794905915392000000*th3dot*sin(th2)*sin(th3) - 795598339977096578581794905915392000000*th1dot*cos(th2)^2*sin(th3) + 795598339977096578581794905915392000000*th2dot*cos(th3)^2*sin(th2) + 795598339977096578581794905915392000000*th2dot*cos(th3)*sin(th2)*sin(th3) + 795598339977096578581794905915392000000*th1dot*cos(th2)*cos(th3)^2*sin(th2) - 795598339977096578581794905915392000000*th1dot*cos(th2)*cos(th3)*sin(th2)*sin(th3))/(140800205444266547517405832452217960942325*cos(th2)), (397799169988548289290897452957696000000*th1dot*sin(2*th2) + 1419410730694772925795933922925238500000*th2dot*sin(th2) - 795598339977096578581794905915392000000*th2dot*cos(th2)*cos(th3) + 795598339977096578581794905915392000000*th2dot*cos(th2)*sin(th3) + 795598339977096578581794905915392000000*th1dot*cos(th2)^2*cos(th3) + 795598339977096578581794905915392000000*th1dot*cos(th2)^2*sin(th3) - 1591196679954193157163589811830784000000*th2dot*cos(th3)*sin(th2)*sin(th3) - 1591196679954193157163589811830784000000*th1dot*cos(th2)*cos(th3)^2*sin(th2))/(140800205444266547517405832452217960942325*cos(th2))
         (68520719092170281189376*sin(th1)*sin(th2)*sin(th3))/1843260477247944264925 - (68520719092170281189376*cos(th2)*sin(th1))/1843260477247944264925 - (68520719092170281189376*cos(th1)*cos(th3))/1843260477247944264925,                                                                                                                                                                                                                                                                                                                                                                                                                                                                                                                                                                                                                                                                                                                                                                                                                                                                                                                                                                                                                                                                                                                                                                                                                                                                                                                                                                                                                                                                                                                                                                                                                                                                                                                                                                                                                                                                                                                                                                                                                                                                                                                                                                                                                                                                                                                                                                                                                                                                                                                                                                                                                                                                                                                                                                                                                                                                                                                                                                                                                                                                                                                                                                                                                                                                                                                                                                                                                                                                                                                                                                                                                                                                                                                                                                                                                                                                                                                                                                                                                                                                                                                                                                                                                                                                                                                                                                                                                                                                                                                                                                                                                                                                                                                                                                                                                                                                                                                                                                                                                                                                                                                                                                                                                                                                                                                                                                                                                                                                                                                                                                                                                                                                                                                                                                                                                                                                                                                                                                                                                                                                                                                                                                                                                                                                                                                                                                                                                                                                                                                                                                                                                                                                                                                                                                                                                                                                                                                                                                                                                                                                                                                                                                                                                                                                                                                                                                                                                                                                                                                                                                                                                                                                                                                                                                                                                                                                                                                                                                                                                                                                                                                                                                                                                                                                                                                                                                                                                                                                                                                                                                                                                                                                                                                                                                                                                                                                                                                                                                                                                                                                                   (31823933599083863143271796236615680000*qxdot*th1dot*cos(th2))/5632008217770661900696233298088718437693 - (68520719092170281189376*cos(th1)*sin(th2))/1843260477247944264925 - (56776429227790917031837356917009540000*qydot*th1dot*cos(th2))/5632008217770661900696233298088718437693 + (194843734278557138944*th1dot*th3dot*cos(th2))/368652095449588852985 - (97421867139278569472*th1dot*th2dot*sin(th2))/368652095449588852985 + (97421867139278569472*th1dot^2*cos(th2)^2*cos(th3))/368652095449588852985 - (97421867139278569472*th1dot^2*cos(th3)*sin(th2)^2)/368652095449588852985 + (389687468557114277888*th1dot^2*cos(th2)*sin(th2))/368652095449588852985 - (68520719092170281189376*cos(th1)*cos(th2)*sin(th3))/1843260477247944264925 - (31823933599083863143271796236615680000*qydot*th1dot*cos(th3)*sin(th2))/5632008217770661900696233298088718437693 + (31823933599083863143271796236615680000*qzdot*th1dot*cos(th3)*sin(th2))/5632008217770661900696233298088718437693 + (97421867139278569472*th1dot*th2dot*cos(th2)*sin(th3))/368652095449588852985 - (97421867139278569472*th1dot*th3dot*cos(th3)*sin(th2))/368652095449588852985 - (31823933599083863143271796236615680000*qxdot*th1dot*sin(th2)*sin(th3))/5632008217770661900696233298088718437693 + (56776429227790917031837356917009540000*qzdot*th1dot*sin(th2)*sin(th3))/5632008217770661900696233298088718437693 - (194843734278557138944*th1dot^2*cos(th2)*cos(th3)^2*sin(th2))/368652095449588852985 + (194843734278557138944*th1dot*th2dot*cos(th3)^2*sin(th2))/368652095449588852985 - (194843734278557138944*th1dot^2*cos(th2)*cos(th3)*sin(th2)*sin(th3))/368652095449588852985 - (194843734278557138944*th1dot*th2dot*cos(th3)*sin(th2)*sin(th3))/368652095449588852985,                                                                                                                                                                                                                                                                                                                                                                                                                                                                                                                                                                                                                                                                                                                                                                                                                                                                                                                                                                                                                                                                                                                                                                                                                                                                                                                                                                                                                                                                                                                                                                                                                                                                                                                                                                                                                                                                                                                                                                                                                                                                                                                                                                                                                                                                                                                                                                                                                                                                                                                                                                                                                                                                                                                                                                                                                                                                                            (68520719092170281189376*sin(th1)*sin(th3))/1843260477247944264925 - (97421867139278569472*th2dot^2*cos(2*th3))/368652095449588852985 + (31823933599083863143271796236615680000*qydot*th2dot*cos(th3))/5632008217770661900696233298088718437693 - (31823933599083863143271796236615680000*qzdot*th2dot*cos(th3))/5632008217770661900696233298088718437693 + (97421867139278569472*th2dot*th3dot*cos(th3))/368652095449588852985 + (31823933599083863143271796236615680000*qxdot*th2dot*sin(th3))/5632008217770661900696233298088718437693 - (56776429227790917031837356917009540000*qzdot*th2dot*sin(th3))/5632008217770661900696233298088718437693 + (97421867139278569472*th1dot^2*cos(th2)^2*cos(th3)^2)/368652095449588852985 - (97421867139278569472*th1dot^2*cos(th2)^2*sin(th3)^2)/368652095449588852985 + (194843734278557138944*th2dot^2*cos(th3)*sin(th3))/368652095449588852985 - (68520719092170281189376*cos(th1)*cos(th3)*sin(th2))/1843260477247944264925 - (31823933599083863143271796236615680000*qydot*th1dot*cos(th2)*sin(th3))/5632008217770661900696233298088718437693 + (31823933599083863143271796236615680000*qzdot*th1dot*cos(th2)*sin(th3))/5632008217770661900696233298088718437693 + (97421867139278569472*th1dot*th2dot*cos(th3)*sin(th2))/368652095449588852985 - (97421867139278569472*th1dot*th3dot*cos(th2)*sin(th3))/368652095449588852985 - (194843734278557138944*th1dot^2*cos(th2)^2*cos(th3)*sin(th3))/368652095449588852985 + (194843734278557138944*th1dot*th2dot*cos(th2)*cos(th3)^2)/368652095449588852985 - (194843734278557138944*th1dot*th2dot*cos(th2)*sin(th3)^2)/368652095449588852985 - (97421867139278569472*th1dot^2*cos(th2)*sin(th2)*sin(th3))/368652095449588852985 + (31823933599083863143271796236615680000*qxdot*th1dot*cos(th2)*cos(th3))/5632008217770661900696233298088718437693 - (56776429227790917031837356917009540000*qzdot*th1dot*cos(th2)*cos(th3))/5632008217770661900696233298088718437693 + (389687468557114277888*th1dot*th2dot*cos(th2)*cos(th3)*sin(th3))/368652095449588852985,                                                                                                                                                                                                                                                                                                                                                                                                                                                                                                                                                                                                                                                                                                                                                                  (194843734278557138944*th1dot)/368652095449588852985 - (389687468557114277888*th1dot*cos(th2)^2)/368652095449588852985 + (97421867139278569472*th2dot*cos(th2))/368652095449588852985 + (31823933599083863143271796236615680000*qxdot*sin(th2))/5632008217770661900696233298088718437693 - (56776429227790917031837356917009540000*qydot*sin(th2))/5632008217770661900696233298088718437693 + (194843734278557138944*th3dot*sin(th2))/368652095449588852985 + (194843734278557138944*th1dot*cos(th2)^2*cos(th3)^2)/368652095449588852985 + (31823933599083863143271796236615680000*qydot*cos(th2)*cos(th3))/5632008217770661900696233298088718437693 - (31823933599083863143271796236615680000*qzdot*cos(th2)*cos(th3))/5632008217770661900696233298088718437693 + (97421867139278569472*th3dot*cos(th2)*cos(th3))/368652095449588852985 + (31823933599083863143271796236615680000*qxdot*cos(th2)*sin(th3))/5632008217770661900696233298088718437693 - (56776429227790917031837356917009540000*qzdot*cos(th2)*sin(th3))/5632008217770661900696233298088718437693 + (97421867139278569472*th2dot*sin(th2)*sin(th3))/368652095449588852985 - (194843734278557138944*th2dot*cos(th2)*cos(th3)^2)/368652095449588852985 + (194843734278557138944*th1dot*cos(th2)*cos(th3)*sin(th2))/368652095449588852985 + (194843734278557138944*th2dot*cos(th2)*cos(th3)*sin(th3))/368652095449588852985 + (194843734278557138944*th1dot*cos(th2)^2*cos(th3)*sin(th3))/368652095449588852985,                                                                                                                                                                                                                                                                                                                                                                                                                                                                                                                                                                                                                                                                                                                                                                                                                                               (56776429227790917031837356917009540000*qzdot*cos(th3))/5632008217770661900696233298088718437693 - (97421867139278569472*th2dot*sin(2*th3))/368652095449588852985 - (31823933599083863143271796236615680000*qxdot*cos(th3))/5632008217770661900696233298088718437693 - (194843734278557138944*th2dot*cos(th3)^2)/368652095449588852985 + (97421867139278569472*th1dot*cos(th2))/368652095449588852985 + (31823933599083863143271796236615680000*qydot*sin(th3))/5632008217770661900696233298088718437693 - (31823933599083863143271796236615680000*qzdot*sin(th3))/5632008217770661900696233298088718437693 + (97421867139278569472*th3dot*sin(th3))/368652095449588852985 + (97421867139278569472*th1dot*sin(th2)*sin(th3))/368652095449588852985 - (194843734278557138944*th1dot*cos(th2)*cos(th3)^2)/368652095449588852985 + (194843734278557138944*th1dot*cos(th2)*cos(th3)*sin(th3))/368652095449588852985,                                                                                                                                                                                                                                                                                                                                                                                                                                                                                                                                                                                                                                                                                                                                                                                                                                                      (31823933599083863143271796236615680000*qxdot)/5632008217770661900696233298088718437693 - (56776429227790917031837356917009540000*qydot)/5632008217770661900696233298088718437693 + (194843734278557138944*th3dot)/368652095449588852985 + (194843734278557138944*th1dot*sin(th2))/368652095449588852985 + (97421867139278569472*th2dot*sin(th3))/368652095449588852985 + (97421867139278569472*th1dot*cos(th2)*cos(th3))/368652095449588852985,                                                                                                                                                                                                                                                                                                                                                                                                                                                                                                                                                                        (31823933599083863143271796236615680000*th3dot)/5632008217770661900696233298088718437693 - (31823933599083863143271796236615680000*th2dot*cos(th3))/5632008217770661900696233298088718437693 + (31823933599083863143271796236615680000*th1dot*sin(th2))/5632008217770661900696233298088718437693 + (31823933599083863143271796236615680000*th1dot*cos(th2)*sin(th3))/5632008217770661900696233298088718437693,                                                                                                                                                                                                                                                                                                                                                                                                                                                                                                                                                               (31823933599083863143271796236615680000*th2dot*sin(th3))/5632008217770661900696233298088718437693 - (56776429227790917031837356917009540000*th1dot*sin(th2))/5632008217770661900696233298088718437693 - (56776429227790917031837356917009540000*th3dot)/5632008217770661900696233298088718437693 + (31823933599083863143271796236615680000*th1dot*cos(th2)*cos(th3))/5632008217770661900696233298088718437693,                                                                                                                                                                                          (56776429227790917031837356917009540000*th2dot*cos(th3))/5632008217770661900696233298088718437693 - (31823933599083863143271796236615680000*th2dot*sin(th3))/5632008217770661900696233298088718437693 - (31823933599083863143271796236615680000*th1dot*cos(th2)*cos(th3))/5632008217770661900696233298088718437693 - (56776429227790917031837356917009540000*th1dot*cos(th2)*sin(th3))/5632008217770661900696233298088718437693
         (68520719092170281189376*cos(th2)*sin(th1))/1843260477247944264925 + (68520719092170281189376*cos(th1)*sin(th3))/1843260477247944264925 + (68520719092170281189376*cos(th3)*sin(th1)*sin(th2))/1843260477247944264925,                                                                                                                                                                                                                                                                                                                                                                                                                                                                                                                                                                                                                                                                                                                                                                                                                                                                                                                                                                                                                                                                                                                                                                                                                                                                                                                                                                                                                                                                                                                                                                                                                                                                                                                                                                                                                                                                                                                                                                                                                                                                                                                                                                                                                                                                                                                                                                                                                                                                                                                                                                                                                                                                                                                                                                                                                                                                                                                                                                                                                                                                                                                                                                                                                                                                                                                                                                                                                                                                                                                                                                                                                                                                                                                                                                                                                                                                                                                                                                                                                                                                                                                                                                                                                                                                                                                                                                                                                                                                                                                                                                                                                                                                                                                                                                                                                                                                                                                                                                                                                                                                                                                                                                                                                                                                                                                                                                                                                                                                                                                                                                                                                                                                                                                                                                                                                                                                                                                                                                                                                                                                                                                                                                                                                                                                                                                                                                                                                                                                                                                                                                                                                                                                                                                                                                                                                                                                                                                                                                                                                                                                                                                                                                                                                                                                                                                                                                                                                                                                                                                                                                                                                                                                                                                                                                                                                                                                                                                                                                                                                                                                                                                                                                                                                                                                                                                                                                                                                                                                                                                                                                                                                                                                                                                                                                                                                                                                                                                                                                                                                                                                                   (68520719092170281189376*cos(th1)*sin(th2))/1843260477247944264925 + (56776429227790917031837356917009540000*qxdot*th1dot*cos(th2))/5632008217770661900696233298088718437693 - (31823933599083863143271796236615680000*qydot*th1dot*cos(th2))/5632008217770661900696233298088718437693 - (194843734278557138944*th1dot*th3dot*cos(th2))/368652095449588852985 + (97421867139278569472*th1dot*th2dot*sin(th2))/368652095449588852985 + (97421867139278569472*th1dot^2*cos(th2)^2*sin(th3))/368652095449588852985 - (97421867139278569472*th1dot^2*sin(th2)^2*sin(th3))/368652095449588852985 - (68520719092170281189376*cos(th1)*cos(th2)*cos(th3))/1843260477247944264925 - (194843734278557138944*th1dot^2*cos(th2)*sin(th2))/368652095449588852985 - (31823933599083863143271796236615680000*qydot*th1dot*cos(th3)*sin(th2))/5632008217770661900696233298088718437693 + (56776429227790917031837356917009540000*qzdot*th1dot*cos(th3)*sin(th2))/5632008217770661900696233298088718437693 - (31823933599083863143271796236615680000*qxdot*th1dot*sin(th2)*sin(th3))/5632008217770661900696233298088718437693 + (31823933599083863143271796236615680000*qzdot*th1dot*sin(th2)*sin(th3))/5632008217770661900696233298088718437693 - (97421867139278569472*th1dot*th3dot*sin(th2)*sin(th3))/368652095449588852985 - (194843734278557138944*th1dot^2*cos(th2)*cos(th3)^2*sin(th2))/368652095449588852985 - (194843734278557138944*th1dot*th2dot*cos(th3)^2*sin(th2))/368652095449588852985 - (97421867139278569472*th1dot*th2dot*cos(th2)*cos(th3))/368652095449588852985 + (194843734278557138944*th1dot^2*cos(th2)*cos(th3)*sin(th2)*sin(th3))/368652095449588852985 - (194843734278557138944*th1dot*th2dot*cos(th3)*sin(th2)*sin(th3))/368652095449588852985,                                                                                                                                                                                                                                                                                                                                                                                                                                                                                                                                                                                                                                                                                                                                                                                                                                                                                                                                                                                                                                                                                                                                                                                                                                                                                                                                                                                                                                                                                                                                                                                                                                                                                                                                                                                                                                                                                                                                                                                                                                                                                                                                                                                                                                                                                                                                                                                                                                                                                                                                                                                                                                                                                                                                                                                                                                                                                            (68520719092170281189376*cos(th3)*sin(th1))/1843260477247944264925 + (97421867139278569472*th2dot^2*cos(2*th3))/368652095449588852985 + (68520719092170281189376*cos(th1)*sin(th2)*sin(th3))/1843260477247944264925 + (31823933599083863143271796236615680000*qydot*th2dot*cos(th3))/5632008217770661900696233298088718437693 - (56776429227790917031837356917009540000*qzdot*th2dot*cos(th3))/5632008217770661900696233298088718437693 + (31823933599083863143271796236615680000*qxdot*th2dot*sin(th3))/5632008217770661900696233298088718437693 - (31823933599083863143271796236615680000*qzdot*th2dot*sin(th3))/5632008217770661900696233298088718437693 + (97421867139278569472*th2dot*th3dot*sin(th3))/368652095449588852985 - (97421867139278569472*th1dot^2*cos(th2)^2*cos(th3)^2)/368652095449588852985 + (97421867139278569472*th1dot^2*cos(th2)^2*sin(th3)^2)/368652095449588852985 + (194843734278557138944*th2dot^2*cos(th3)*sin(th3))/368652095449588852985 - (31823933599083863143271796236615680000*qydot*th1dot*cos(th2)*sin(th3))/5632008217770661900696233298088718437693 + (56776429227790917031837356917009540000*qzdot*th1dot*cos(th2)*sin(th3))/5632008217770661900696233298088718437693 + (97421867139278569472*th1dot*th2dot*sin(th2)*sin(th3))/368652095449588852985 - (194843734278557138944*th1dot^2*cos(th2)^2*cos(th3)*sin(th3))/368652095449588852985 + (194843734278557138944*th1dot*th2dot*cos(th2)*cos(th3)^2)/368652095449588852985 - (194843734278557138944*th1dot*th2dot*cos(th2)*sin(th3)^2)/368652095449588852985 + (97421867139278569472*th1dot^2*cos(th2)*cos(th3)*sin(th2))/368652095449588852985 + (31823933599083863143271796236615680000*qxdot*th1dot*cos(th2)*cos(th3))/5632008217770661900696233298088718437693 - (31823933599083863143271796236615680000*qzdot*th1dot*cos(th2)*cos(th3))/5632008217770661900696233298088718437693 + (97421867139278569472*th1dot*th3dot*cos(th2)*cos(th3))/368652095449588852985 - (389687468557114277888*th1dot*th2dot*cos(th2)*cos(th3)*sin(th3))/368652095449588852985,                                                                                                                                                                                                                                                                                                                                                                                                                                                                                                                                                                                                                                                                                                                                                                  (194843734278557138944*th1dot*cos(th2)^2)/368652095449588852985 - (194843734278557138944*th1dot)/368652095449588852985 - (97421867139278569472*th2dot*cos(th2))/368652095449588852985 + (56776429227790917031837356917009540000*qxdot*sin(th2))/5632008217770661900696233298088718437693 - (31823933599083863143271796236615680000*qydot*sin(th2))/5632008217770661900696233298088718437693 - (194843734278557138944*th3dot*sin(th2))/368652095449588852985 + (194843734278557138944*th1dot*cos(th2)^2*cos(th3)^2)/368652095449588852985 + (31823933599083863143271796236615680000*qydot*cos(th2)*cos(th3))/5632008217770661900696233298088718437693 - (56776429227790917031837356917009540000*qzdot*cos(th2)*cos(th3))/5632008217770661900696233298088718437693 + (31823933599083863143271796236615680000*qxdot*cos(th2)*sin(th3))/5632008217770661900696233298088718437693 - (31823933599083863143271796236615680000*qzdot*cos(th2)*sin(th3))/5632008217770661900696233298088718437693 - (97421867139278569472*th2dot*cos(th3)*sin(th2))/368652095449588852985 + (97421867139278569472*th3dot*cos(th2)*sin(th3))/368652095449588852985 + (194843734278557138944*th2dot*cos(th2)*cos(th3)^2)/368652095449588852985 + (194843734278557138944*th2dot*cos(th2)*cos(th3)*sin(th3))/368652095449588852985 + (194843734278557138944*th1dot*cos(th2)*sin(th2)*sin(th3))/368652095449588852985 - (194843734278557138944*th1dot*cos(th2)^2*cos(th3)*sin(th3))/368652095449588852985,                                                                                                                                                                                                                                                                                                                                                                                                                                                                                                                                                                                                                                                                                                                                                                                        (194843734278557138944*th2dot)/368652095449588852985 - (194843734278557138944*th2dot*cos(th3)^2)/368652095449588852985 + (97421867139278569472*th2dot*sin(2*th3))/368652095449588852985 - (31823933599083863143271796236615680000*qxdot*cos(th3))/5632008217770661900696233298088718437693 + (31823933599083863143271796236615680000*qzdot*cos(th3))/5632008217770661900696233298088718437693 - (97421867139278569472*th1dot*cos(th2))/368652095449588852985 - (97421867139278569472*th3dot*cos(th3))/368652095449588852985 + (31823933599083863143271796236615680000*qydot*sin(th3))/5632008217770661900696233298088718437693 - (56776429227790917031837356917009540000*qzdot*sin(th3))/5632008217770661900696233298088718437693 - (97421867139278569472*th1dot*cos(th3)*sin(th2))/368652095449588852985 + (194843734278557138944*th1dot*cos(th2)*cos(th3)^2)/368652095449588852985 + (194843734278557138944*th1dot*cos(th2)*cos(th3)*sin(th3))/368652095449588852985,                                                                                                                                                                                                                                                                                                                                                                                                                                                                                                                                                                                                                                                                                                                                                                                                                                                      (56776429227790917031837356917009540000*qxdot)/5632008217770661900696233298088718437693 - (31823933599083863143271796236615680000*qydot)/5632008217770661900696233298088718437693 - (194843734278557138944*th3dot)/368652095449588852985 - (97421867139278569472*th2dot*cos(th3))/368652095449588852985 - (194843734278557138944*th1dot*sin(th2))/368652095449588852985 + (97421867139278569472*th1dot*cos(th2)*sin(th3))/368652095449588852985,                                                                                                                                                                                                                                                                                                                                                                                                                                                                                                                                                                        (56776429227790917031837356917009540000*th3dot)/5632008217770661900696233298088718437693 - (31823933599083863143271796236615680000*th2dot*cos(th3))/5632008217770661900696233298088718437693 + (56776429227790917031837356917009540000*th1dot*sin(th2))/5632008217770661900696233298088718437693 + (31823933599083863143271796236615680000*th1dot*cos(th2)*sin(th3))/5632008217770661900696233298088718437693,                                                                                                                                                                                                                                                                                                                                                                                                                                                                                                                                                               (31823933599083863143271796236615680000*th2dot*sin(th3))/5632008217770661900696233298088718437693 - (31823933599083863143271796236615680000*th1dot*sin(th2))/5632008217770661900696233298088718437693 - (31823933599083863143271796236615680000*th3dot)/5632008217770661900696233298088718437693 + (31823933599083863143271796236615680000*th1dot*cos(th2)*cos(th3))/5632008217770661900696233298088718437693,                                                                                                                                                                                          (31823933599083863143271796236615680000*th2dot*cos(th3))/5632008217770661900696233298088718437693 - (56776429227790917031837356917009540000*th2dot*sin(th3))/5632008217770661900696233298088718437693 - (56776429227790917031837356917009540000*th1dot*cos(th2)*cos(th3))/5632008217770661900696233298088718437693 - (31823933599083863143271796236615680000*th1dot*cos(th2)*sin(th3))/5632008217770661900696233298088718437693
         (68520719092170281189376*cos(th1)*cos(th3))/1843260477247944264925 - (68520719092170281189376*cos(th1)*sin(th3))/1843260477247944264925 - (68520719092170281189376*cos(th3)*sin(th1)*sin(th2))/1843260477247944264925 - (68520719092170281189376*sin(th1)*sin(th2)*sin(th3))/1843260477247944264925,                                                                                                                                                                                                                                                                                                                                                                                                                                                                                                                                                                                                                                                                                                                                                                                                                                                                                                                                                                                                                                                                                                                                                                                                                                                                                                                                                                                                                                                                                                                                                                                                                                                                                                                                                                                                                                                                                                                                                                                                                                                                                                                                                                                                                                                                                                                                                                                                                                                                                                                                                                                                                                                                                                                                                                                                                                                                                                                                                                                                                                                                                                                                                                                                                                                                                                                                                                                                                                                                                                                                                                                                                                                                                                                                                                                                                                                                                                                                                                                                                                                                                                                                                                                                                                                                                                                                                                                                                                                                                                                                                                                                                                                                                                                                                                                                                                                                                                                                                                                                                                                                                                                                                                                                                                                                                                                                                                                                                                                                                                                                                                                                                                                                                                                                                                                                                                                                                                                                                                                                                                                                                                                                                                                                                                                                                                                                                                                                                                                                                                                                                                                                                                                                                                                                                                                                                                                                                                                                                                                                                                                                                                                                                                                                                                                                                                                                                                                                                                                                                                                                                                                                                                                                                                                                                                                                                                                                                                                                                                                                                                                                                                                                                                                                                                                                                                                                                                                                                                                                                                                                                                                                                                                                                                                                                                                                                                                                                                                                                                                                                                                                                (31823933599083863143271796236615680000*qxdot*th1dot*cos(th2))/5632008217770661900696233298088718437693 - (31823933599083863143271796236615680000*qydot*th1dot*cos(th2))/5632008217770661900696233298088718437693 - (97421867139278569472*th1dot^2*cos(th2)^2*cos(th3))/368652095449588852985 + (97421867139278569472*th1dot^2*cos(th3)*sin(th2)^2)/368652095449588852985 - (97421867139278569472*th1dot^2*cos(th2)^2*sin(th3))/368652095449588852985 + (97421867139278569472*th1dot^2*sin(th2)^2*sin(th3))/368652095449588852985 + (68520719092170281189376*cos(th1)*cos(th2)*cos(th3))/1843260477247944264925 - (194843734278557138944*th1dot^2*cos(th2)*sin(th2))/368652095449588852985 + (68520719092170281189376*cos(th1)*cos(th2)*sin(th3))/1843260477247944264925 - (56776429227790917031837356917009540000*qydot*th1dot*cos(th3)*sin(th2))/5632008217770661900696233298088718437693 + (31823933599083863143271796236615680000*qzdot*th1dot*cos(th3)*sin(th2))/5632008217770661900696233298088718437693 - (97421867139278569472*th1dot*th2dot*cos(th2)*sin(th3))/368652095449588852985 + (97421867139278569472*th1dot*th3dot*cos(th3)*sin(th2))/368652095449588852985 - (56776429227790917031837356917009540000*qxdot*th1dot*sin(th2)*sin(th3))/5632008217770661900696233298088718437693 + (31823933599083863143271796236615680000*qzdot*th1dot*sin(th2)*sin(th3))/5632008217770661900696233298088718437693 + (97421867139278569472*th1dot*th3dot*sin(th2)*sin(th3))/368652095449588852985 + (389687468557114277888*th1dot^2*cos(th2)*cos(th3)^2*sin(th2))/368652095449588852985 + (97421867139278569472*th1dot*th2dot*cos(th2)*cos(th3))/368652095449588852985 + (389687468557114277888*th1dot*th2dot*cos(th3)*sin(th2)*sin(th3))/368652095449588852985,                                                                                                                                                                                                                                                                                                                                                                                                                                                                                                                                                                                                                                                                                                                                                                                                                                                                                                                                                                                                                                                                                                                                                                                                                                                                                                                                                                                                                                                                                                                                                                                                                                                                                                                                                                                                                                                                                                                                                                                                                                                                                                                                                                                                                                                                                                                                                                                                                                                                                                                                                                                                                                                                                                                                          (56776429227790917031837356917009540000*qydot*th2dot*cos(th3))/5632008217770661900696233298088718437693 - (68520719092170281189376*sin(th1)*sin(th3))/1843260477247944264925 - (68520719092170281189376*cos(th1)*sin(th2)*sin(th3))/1843260477247944264925 - (68520719092170281189376*cos(th3)*sin(th1))/1843260477247944264925 - (31823933599083863143271796236615680000*qzdot*th2dot*cos(th3))/5632008217770661900696233298088718437693 - (97421867139278569472*th2dot*th3dot*cos(th3))/368652095449588852985 + (56776429227790917031837356917009540000*qxdot*th2dot*sin(th3))/5632008217770661900696233298088718437693 - (31823933599083863143271796236615680000*qzdot*th2dot*sin(th3))/5632008217770661900696233298088718437693 - (97421867139278569472*th2dot*th3dot*sin(th3))/368652095449588852985 - (389687468557114277888*th2dot^2*cos(th3)*sin(th3))/368652095449588852985 + (68520719092170281189376*cos(th1)*cos(th3)*sin(th2))/1843260477247944264925 - (56776429227790917031837356917009540000*qydot*th1dot*cos(th2)*sin(th3))/5632008217770661900696233298088718437693 + (31823933599083863143271796236615680000*qzdot*th1dot*cos(th2)*sin(th3))/5632008217770661900696233298088718437693 - (97421867139278569472*th1dot*th2dot*cos(th3)*sin(th2))/368652095449588852985 + (97421867139278569472*th1dot*th3dot*cos(th2)*sin(th3))/368652095449588852985 - (97421867139278569472*th1dot*th2dot*sin(th2)*sin(th3))/368652095449588852985 + (389687468557114277888*th1dot^2*cos(th2)^2*cos(th3)*sin(th3))/368652095449588852985 - (389687468557114277888*th1dot*th2dot*cos(th2)*cos(th3)^2)/368652095449588852985 + (389687468557114277888*th1dot*th2dot*cos(th2)*sin(th3)^2)/368652095449588852985 - (97421867139278569472*th1dot^2*cos(th2)*cos(th3)*sin(th2))/368652095449588852985 + (97421867139278569472*th1dot^2*cos(th2)*sin(th2)*sin(th3))/368652095449588852985 + (56776429227790917031837356917009540000*qxdot*th1dot*cos(th2)*cos(th3))/5632008217770661900696233298088718437693 - (31823933599083863143271796236615680000*qzdot*th1dot*cos(th2)*cos(th3))/5632008217770661900696233298088718437693 - (97421867139278569472*th1dot*th3dot*cos(th2)*cos(th3))/368652095449588852985,                                                                                                                                                                                                                                                                                                                                                                                                                                                                                                                                                                                                                                                                                                                                                                                                                                                                                     (194843734278557138944*th1dot*cos(th2)^2)/368652095449588852985 + (31823933599083863143271796236615680000*qxdot*sin(th2))/5632008217770661900696233298088718437693 - (31823933599083863143271796236615680000*qydot*sin(th2))/5632008217770661900696233298088718437693 - (389687468557114277888*th1dot*cos(th2)^2*cos(th3)^2)/368652095449588852985 + (56776429227790917031837356917009540000*qydot*cos(th2)*cos(th3))/5632008217770661900696233298088718437693 - (31823933599083863143271796236615680000*qzdot*cos(th2)*cos(th3))/5632008217770661900696233298088718437693 - (97421867139278569472*th3dot*cos(th2)*cos(th3))/368652095449588852985 + (56776429227790917031837356917009540000*qxdot*cos(th2)*sin(th3))/5632008217770661900696233298088718437693 - (31823933599083863143271796236615680000*qzdot*cos(th2)*sin(th3))/5632008217770661900696233298088718437693 + (97421867139278569472*th2dot*cos(th3)*sin(th2))/368652095449588852985 - (97421867139278569472*th3dot*cos(th2)*sin(th3))/368652095449588852985 - (97421867139278569472*th2dot*sin(th2)*sin(th3))/368652095449588852985 - (194843734278557138944*th1dot*cos(th2)*cos(th3)*sin(th2))/368652095449588852985 - (389687468557114277888*th2dot*cos(th2)*cos(th3)*sin(th3))/368652095449588852985 - (194843734278557138944*th1dot*cos(th2)*sin(th2)*sin(th3))/368652095449588852985,                                                                                                                                                                                                                                                                                                                                                                                                                                                                                                                                                                                                                                                                                                                                                                                                                                                            (389687468557114277888*th2dot*cos(th3)^2)/368652095449588852985 - (194843734278557138944*th2dot)/368652095449588852985 - (56776429227790917031837356917009540000*qxdot*cos(th3))/5632008217770661900696233298088718437693 + (31823933599083863143271796236615680000*qzdot*cos(th3))/5632008217770661900696233298088718437693 + (97421867139278569472*th3dot*cos(th3))/368652095449588852985 + (56776429227790917031837356917009540000*qydot*sin(th3))/5632008217770661900696233298088718437693 - (31823933599083863143271796236615680000*qzdot*sin(th3))/5632008217770661900696233298088718437693 - (97421867139278569472*th3dot*sin(th3))/368652095449588852985 + (97421867139278569472*th1dot*cos(th3)*sin(th2))/368652095449588852985 - (97421867139278569472*th1dot*sin(th2)*sin(th3))/368652095449588852985 - (389687468557114277888*th1dot*cos(th2)*cos(th3)*sin(th3))/368652095449588852985,                                                                                                                                                                                                                                                                                                                                                                                                                                                                                                                                                                                                                                                                                                                                                                                                                                      (31823933599083863143271796236615680000*qxdot)/5632008217770661900696233298088718437693 - (31823933599083863143271796236615680000*qydot)/5632008217770661900696233298088718437693 + (97421867139278569472*th2dot*cos(th3))/368652095449588852985 - (97421867139278569472*th2dot*sin(th3))/368652095449588852985 - (97421867139278569472*th1dot*cos(th2)*cos(th3))/368652095449588852985 - (97421867139278569472*th1dot*cos(th2)*sin(th3))/368652095449588852985,                                                                                                                                                                                                                                                                                                                                                                                                                                                                                                                                                                        (31823933599083863143271796236615680000*th3dot)/5632008217770661900696233298088718437693 - (56776429227790917031837356917009540000*th2dot*cos(th3))/5632008217770661900696233298088718437693 + (31823933599083863143271796236615680000*th1dot*sin(th2))/5632008217770661900696233298088718437693 + (56776429227790917031837356917009540000*th1dot*cos(th2)*sin(th3))/5632008217770661900696233298088718437693,                                                                                                                                                                                                                                                                                                                                                                                                                                                                                                                                                               (56776429227790917031837356917009540000*th2dot*sin(th3))/5632008217770661900696233298088718437693 - (31823933599083863143271796236615680000*th1dot*sin(th2))/5632008217770661900696233298088718437693 - (31823933599083863143271796236615680000*th3dot)/5632008217770661900696233298088718437693 + (56776429227790917031837356917009540000*th1dot*cos(th2)*cos(th3))/5632008217770661900696233298088718437693,                                                                                                                                                                                          (31823933599083863143271796236615680000*th2dot*cos(th3))/5632008217770661900696233298088718437693 - (31823933599083863143271796236615680000*th2dot*sin(th3))/5632008217770661900696233298088718437693 - (31823933599083863143271796236615680000*th1dot*cos(th2)*cos(th3))/5632008217770661900696233298088718437693 - (31823933599083863143271796236615680000*th1dot*cos(th2)*sin(th3))/5632008217770661900696233298088718437693
        ];

    B = [
         0, 0, 0
         0, 0, 0
         0, 0, 0
